simulink model "exp1_p2_3A"  (R2018a)
settings: Solver=VariableStepAuto  StartTime=0.0  StopTime=10.0  RelTol=1e-3
settings Model: Creator=Administrator  LastModifiedBy=Administrator

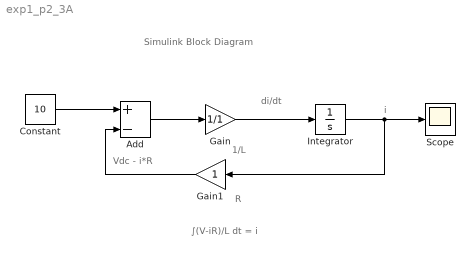
== system exp1_p2_3A ==
  note: Simulink Block Diagram
  note: ∫(V-iR)/L dt = i
  note: di/dt
  note: Vdc - i*R
  note: i
  note: 1/L
  note: R
  Add : Sum  Inputs=+-
  Constant : Constant  Value=10
  Gain : Gain  Gain=1/1
  Gain1 : Gain
  Integrator : Integrator
  Scope : Scope
  wires:
  Constant/1 -> Add/1
  Add/1 -> Gain/1
  Gain/1 -> Integrator/1
  Integrator/1 -> Gain1/1, Scope/1
  Gain1/1 -> Add/2
